simulink model "Final_Model"  (R2013a)
settings: Solver=ode45  StartTime=0.0  StopTime=10.0  RelTol=1e-3
libraries: simulink x47, fuzblock x1
settings Model: Creator=Admin  LastModifiedBy=Admin

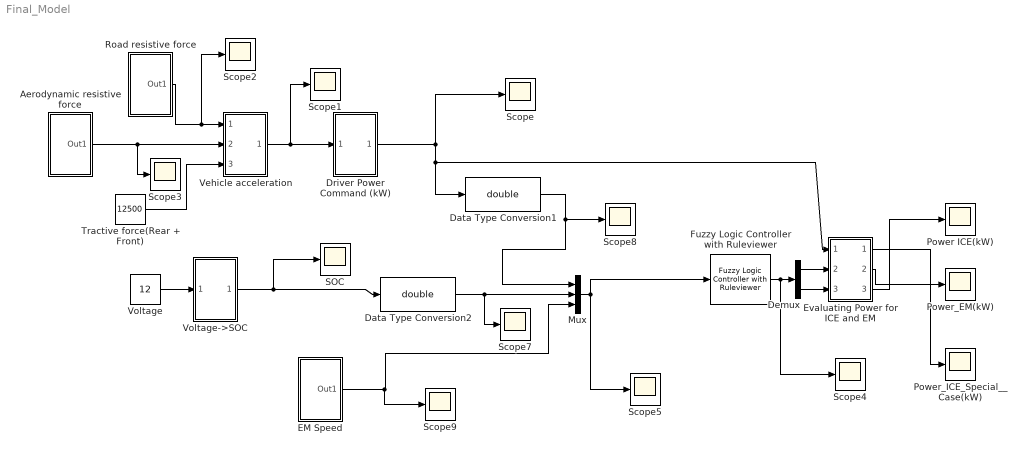
== system Final_Model ==
  Aerodynamic resistive force : Subsystem
  Data Type Conversion1 : DataTypeConversion  OutDataTypeStr=double
  Data Type Conversion2 : DataTypeConversion  OutDataTypeStr=double
  Demux : Demux  Outputs=2
  Driver Power Command (kW) : Subsystem
  EM Speed : Subsystem
  Evaluating Power for ICE and EM : Subsystem
  Fuzzy Logic Controller with Ruleviewer : fuzblock/Fuzzy Logic  Controller  with Ruleviewer  fismatrix=Fuzzy_Controller  Ts=2
  Mux : Mux  Inputs=3
  Power ICE(kW) : Scope
  Power_EM(kW) : Scope
      settings: SaveName=ScopeData6
  Power_ICE_Special__Case(kW) : Scope
      settings: SaveName=ScopeData7
  Road resistive force : Subsystem
  "SOC " : Scope
      settings: SaveName=ScopeData4
  Scope{,1..5,7..9} (9 alike) : Scope
      Scope settings: SaveName=ScopeData5
      Scope1 settings: SaveName=ScopeData8
      Scope2 settings: SaveName=ScopeData9
      Scope3 settings: SaveName=ScopeData10
      Scope4 settings: SaveName=ScopeData11
      Scope5 settings: SaveName=ScopeData2
      Scope7 settings: SaveName=ScopeData14
      Scope8 settings: SaveName=ScopeData15
      Scope9 settings: SaveName=ScopeData3
  Tractive force(Rear + Front) : Constant  Value=12500
  Vehicle acceleration : Subsystem
  Voltage : Constant  Value=12
  Voltage->SOC : Subsystem
  wires:
  Road resistive force/1(Out1) -> Scope2/1, Vehicle acceleration/1(In1)
  Aerodynamic resistive force/1(Out1) -> Scope3/1, Vehicle acceleration/2(In2)
  Tractive force(Rear + Front)/1 -> Vehicle acceleration/3(In3)
  Driver Power Command (kW)/1(Out1) -> Evaluating Power for ICE and EM/1(In1), Data Type Conversion1/1, Scope/1
  EM Speed/1(Out1) -> Scope9/1, Mux/3
  Voltage/1 -> Voltage->SOC/1(In1)
  Fuzzy Logic Controller with Ruleviewer/1 -> Scope4/1, Demux/1
  Mux/1 -> Scope5/1, Fuzzy Logic Controller with Ruleviewer/1
  Data Type Conversion1/1 -> Mux/1, Scope8/1
  Data Type Conversion2/1 -> Scope7/1, Mux/2
  Demux/1 -> Evaluating Power for ICE and EM/2(In2)
  Demux/2 -> Evaluating Power for ICE and EM/3(In3)
  Evaluating Power for ICE and EM/1(Out1) -> Power_ICE_Special__Case(kW)/1
  Evaluating Power for ICE and EM/2(Out2) -> Power_EM(kW)/1
  Voltage->SOC/1(Out1) -> Data Type Conversion2/1, "SOC "/1
  Evaluating Power for ICE and EM/3(Out3) -> Power ICE(kW)/1
  Vehicle acceleration/1(Out1) -> Scope1/1, Driver Power Command (kW)/1(In1)

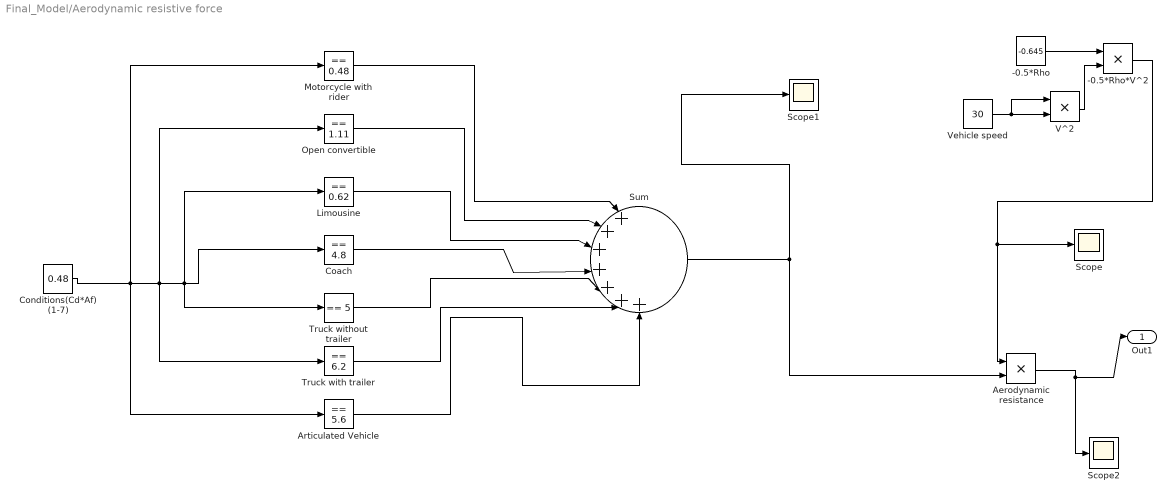
== system Final_Model/Aerodynamic resistive force ==
  -0.5*Rho : Constant  Value=-0.645
  -0.5*Rho*V^2 : Product  RndMeth=Zero
  Aerodynamic resistance : Product  RndMeth=Zero
  Articulated Vehicle : simulink/Logic and Bit Operations/Compare To Constant  relop===  const=5.6  OutDataTypeStr=uint8
  Coach : simulink/Logic and Bit Operations/Compare To Constant  relop===  const=4.8  OutDataTypeStr=uint8
  Conditions(Cd*Af) (1-7) : Constant  Value=0.48
  Limousine : simulink/Logic and Bit Operations/Compare To Constant  relop===  const=0.62  OutDataTypeStr=uint8
  "Motorcycle with rider " : simulink/Logic and Bit Operations/Compare To Constant  relop===  const=0.48  OutDataTypeStr=uint8
  Open convertible : simulink/Logic and Bit Operations/Compare To Constant  relop===  const=1.11  OutDataTypeStr=uint8
  Scope : Scope
      settings: SaveName=ScopeData12
  Scope1 : Scope
      settings: SaveName=ScopeData16
  Scope2 : Scope
      settings: SaveName=ScopeData17
  Sum : Sum  Inputs=|+++++++
  Truck with trailer : simulink/Logic and Bit Operations/Compare To Constant  relop===  const=6.2  OutDataTypeStr=uint8
  Truck without trailer : simulink/Logic and Bit Operations/Compare To Constant  relop===  const=5  OutDataTypeStr=uint8
  V^2 : Product  RndMeth=Zero
  Vehicle speed : Constant  Value=30
  Out1 : Outport
  wires:
  Sum/1 -> Aerodynamic resistance/2, Scope1/1
  Aerodynamic resistance/1 -> Scope2/1, Out1/1
  -0.5*Rho*V^2/1 -> Aerodynamic resistance/1, Scope/1
  V^2/1 -> -0.5*Rho*V^2/2
  -0.5*Rho/1 -> -0.5*Rho*V^2/1
  Conditions(Cd*Af) (1-7)/1 -> "Motorcycle with rider "/1, Articulated Vehicle/1, Open convertible/1, Truck with trailer/1, Limousine/1, Truck without trailer/1, Coach/1
  Truck without trailer/1 -> Sum/5
  Truck with trailer/1 -> Sum/6
  Articulated Vehicle/1 -> Sum/7
  Coach/1 -> Sum/4
  Limousine/1 -> Sum/3
  Open convertible/1 -> Sum/2
  "Motorcycle with rider "/1 -> Sum/1
  Vehicle speed/1 -> V^2/1, V^2/2

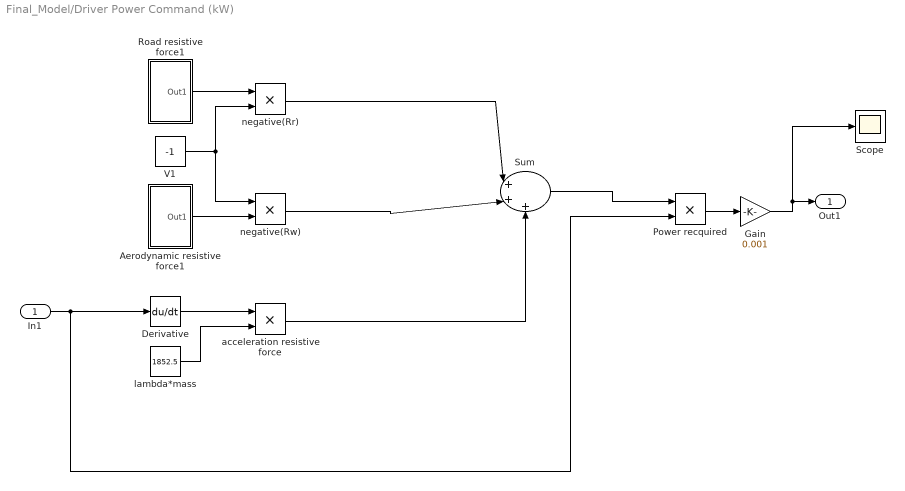
== system Final_Model/Driver Power Command (kW) ==
  In1 : Inport
  Aerodynamic resistive force1 : Subsystem
  Derivative : Derivative
  Gain : Gain  Gain=0.001
  Power recquired : Product  OutDataTypeStr=double  RndMeth=Zero
  Road resistive force1 : Subsystem
  Scope : Scope
      settings: SaveName=ScopeData25
  Sum : Sum  Inputs=|+++  SampleTime=2
  V1 : Constant  Value=-1
  acceleration resistive force : Product  RndMeth=Zero
  lambda*mass : Constant  Value=1852.5
  negative(Rr) : Product  RndMeth=Zero
  negative(Rw) : Product  RndMeth=Zero
  Out1 : Outport
  wires:
  In1/1 -> Power recquired/2, Derivative/1
  Derivative/1 -> acceleration resistive force/1
  lambda*mass/1 -> acceleration resistive force/2
  Road resistive force1/1(Out1) -> negative(Rr)/1
  V1/1 -> negative(Rw)/1, negative(Rr)/2
  Aerodynamic resistive force1/1(Out1) -> negative(Rw)/2
  acceleration resistive force/1 -> Sum/3
  negative(Rw)/1 -> Sum/2
  negative(Rr)/1 -> Sum/1
  Sum/1 -> Power recquired/1
  Power recquired/1 -> Gain/1
  Gain/1 -> Scope/1, Out1/1

== system Final_Model/EM Speed ==
  DC motor : Subsystem
  Out1 : Outport
  wires:
  DC motor/1(Out1) -> Out1/1

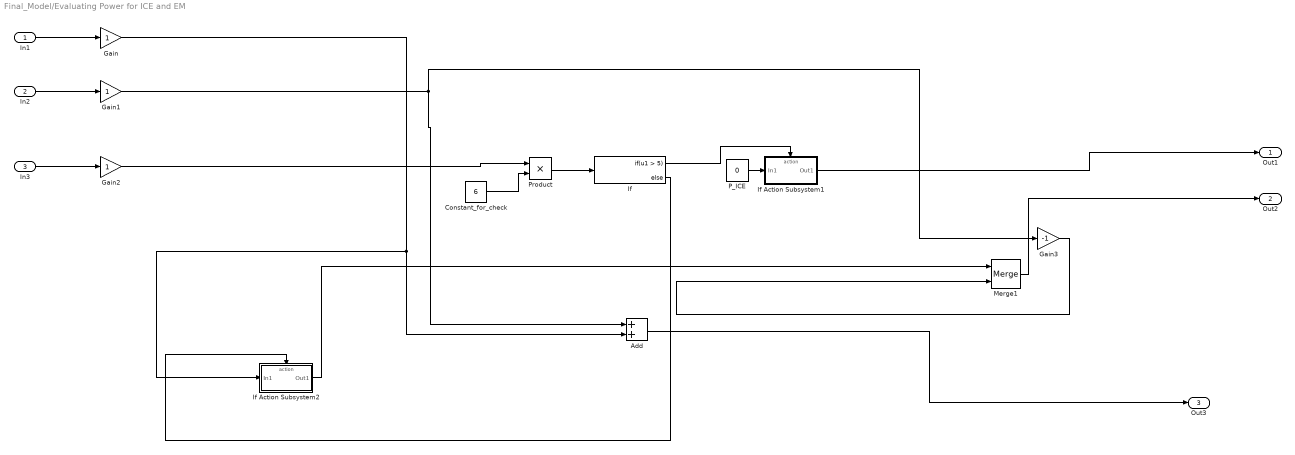
== system Final_Model/Evaluating Power for ICE and EM ==
  In1 : Inport
  In2 : Inport  Port=2
  In3 : Inport  Port=3
  Add : Sum
  Constant_for_check : Constant  Value=6
  Gain : Gain
  Gain1 : Gain
  Gain2 : Gain
  Gain3 : Gain  Gain=-1
  If : If  IfExpression=u1 > 5
  If Action Subsystem1 : Subsystem  TreatAsAtomicUnit=on
  If Action Subsystem2 : Subsystem  TreatAsAtomicUnit=on
  Merge1 : Merge
  P_ICE : Constant  Value=0
  Product : Product
  Out1 : Outport
  Out2 : Outport  Port=2
  Out3 : Outport  Port=3
  wires:
  Merge1/1 -> Out2/1
  Gain3/1 -> Merge1/2
  P_ICE/1 -> If Action Subsystem1/1(In1)
  If/1 -> If Action Subsystem1/Action
  If/2 -> If Action Subsystem2/Action
  Gain/1 -> Add/2, If Action Subsystem2/1(In1)
  In2/1 -> Gain1/1
  In3/1 -> Gain2/1
  Gain2/1 -> Product/1
  Constant_for_check/1 -> Product/2
  Gain1/1 -> Add/1, Gain3/1
  If Action Subsystem2/1(Out1) -> Merge1/1
  In1/1 -> Gain/1
  Product/1 -> If/1
  If Action Subsystem1/1(Out1) -> Out1/1
  Add/1 -> Out3/1

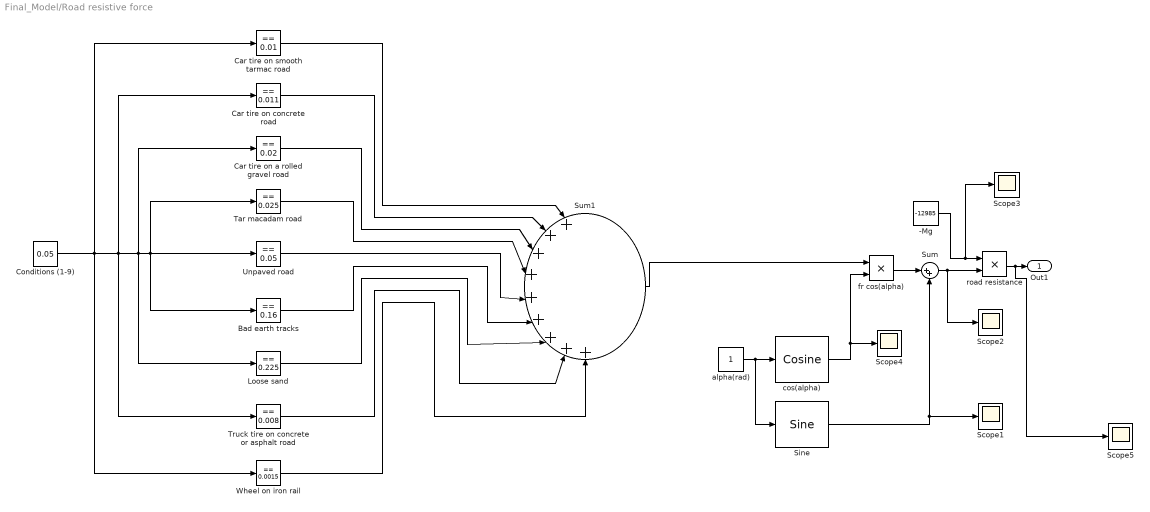
== system Final_Model/Road resistive force ==
  "-Mg " : Constant  Value=-12985
  Bad earth tracks : simulink/Logic and Bit Operations/Compare To Constant  relop===  const=0.16  OutDataTypeStr=uint8
  "Car tire on a rolled gravel road " : simulink/Logic and Bit Operations/Compare To Constant  relop===  const=0.02  OutDataTypeStr=uint8
  Car tire on concrete road : simulink/Logic and Bit Operations/Compare To Constant  relop===  const=0.011  OutDataTypeStr=uint8
  "Car tire on smooth tarmac road " : simulink/Logic and Bit Operations/Compare To Constant  relop===  const=0.01  OutDataTypeStr=uint8
  Conditions (1-9) : Constant  Value=0.05
  Loose sand : simulink/Logic and Bit Operations/Compare To Constant  relop===  const=0.225  OutDataTypeStr=uint8
  Scope{1..5} (5 alike) : Scope
      Scope1 settings: SaveName=ScopeData18
      Scope2 settings: SaveName=ScopeData19
      Scope3 settings: SaveName=ScopeData20
      Scope4 settings: SaveName=ScopeData21
      Scope5 settings: SaveName=ScopeData22
  Sine : simulink/Lookup Tables/Sine  Formula=sin(2*pi*u)  NumDataPoints=(2^5)+1  OutputWordLength=16
  Sum : Sum  Inputs=|++
  Sum1 : Sum  Inputs=|+++++++++
  Tar macadam road : simulink/Logic and Bit Operations/Compare To Constant  relop===  const=0.025  OutDataTypeStr=uint8
  Truck tire on concrete or asphalt road : simulink/Logic and Bit Operations/Compare To Constant  relop===  const=0.008  OutDataTypeStr=uint8
  Unpaved road : simulink/Logic and Bit Operations/Compare To Constant  relop===  const=0.05  OutDataTypeStr=uint8
  Wheel on iron rail : simulink/Logic and Bit Operations/Compare To Constant  relop===  const=0.0015  OutDataTypeStr=uint8
  alpha(rad) : Constant
  cos(alpha) : simulink/Lookup Tables/Cosine  Formula=cos(2*pi*u)  NumDataPoints=(2^5)+1  OutputWordLength=16
  fr cos(alpha) : Product  RndMeth=Zero
  road resistance : Product  RndMeth=Zero
  Out1 : Outport
  wires:
  road resistance/1 -> Scope5/1, Out1/1
  "-Mg "/1 -> Scope3/1, road resistance/1
  Sum/1 -> Scope2/1, road resistance/2
  Sine/1 -> Scope1/1, Sum/2
  fr cos(alpha)/1 -> Sum/1
  alpha(rad)/1 -> Sine/1, cos(alpha)/1
  Sum1/1 -> fr cos(alpha)/1
  cos(alpha)/1 -> Scope4/1, fr cos(alpha)/2
  "Car tire on smooth tarmac road "/1 -> Sum1/1
  Car tire on concrete road/1 -> Sum1/2
  "Car tire on a rolled gravel road "/1 -> Sum1/3
  Tar macadam road/1 -> Sum1/4
  Wheel on iron rail/1 -> Sum1/9
  Truck tire on concrete or asphalt road/1 -> Sum1/8
  Loose sand/1 -> Sum1/7
  Bad earth tracks/1 -> Sum1/6
  Unpaved road/1 -> Sum1/5
  Conditions (1-9)/1 -> Wheel on iron rail/1, Truck tire on concrete or asphalt road/1, Loose sand/1, Bad earth tracks/1, Tar macadam road/1, Unpaved road/1, "Car tire on a rolled gravel road "/1, Car tire on concrete road/1, "Car tire on smooth tarmac road "/1

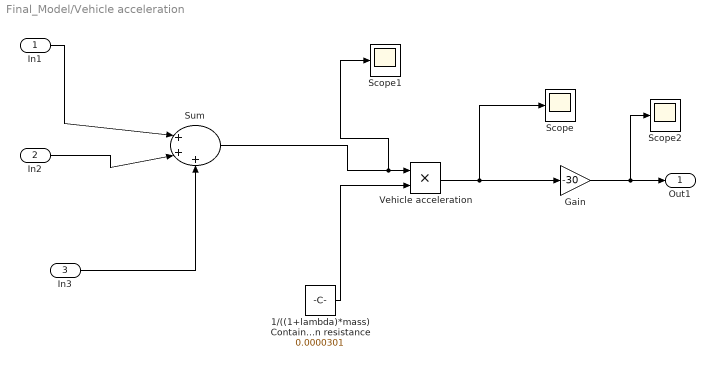
== system Final_Model/Vehicle acceleration ==
  In1 : Inport
  In2 : Inport  Port=2
  In3 : Inport  Port=3
  1/((1+lambda)*mass) Contains acceleration resistance : Constant  Value=0.0000301
  Gain : Gain  Gain=-30
  Scope : Scope
  Scope1 : Scope
      settings: SaveName=ScopeData23
  Scope2 : Scope
      settings: SaveName=ScopeData24
  Sum : Sum  Inputs=|+++
  Vehicle acceleration : Product  RndMeth=Zero
  Out1 : Outport
  wires:
  In1/1 -> Sum/1
  In2/1 -> Sum/2
  In3/1 -> Sum/3
  Sum/1 -> Scope1/1, Vehicle acceleration/1
  1/((1+lambda)*mass) Contains acceleration resistance/1 -> Vehicle acceleration/2
  Vehicle acceleration/1 -> Gain/1, Scope/1
  Gain/1 -> Scope2/1, Out1/1

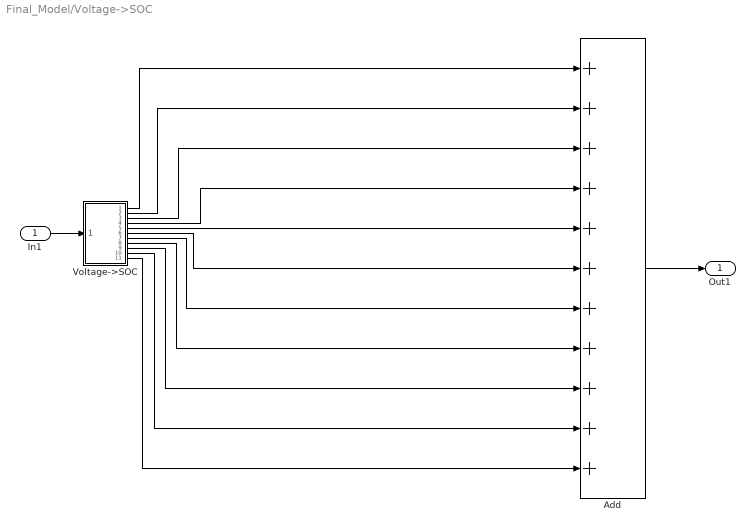
== system Final_Model/Voltage->SOC ==
  In1 : Inport
  Add : Sum  Inputs=+++++++++++  AccumDataTypeStr=uint16  OutDataTypeStr=uint16
  Voltage->SOC : Subsystem
  Out1 : Outport  OutDataTypeStr=uint16
  wires:
  In1/1 -> Voltage->SOC/1(In1)
  Voltage->SOC/1(Out1) -> Add/1
  Voltage->SOC/3(Out3) -> Add/3
  Voltage->SOC/2(Out2) -> Add/2
  Voltage->SOC/10(Out10) -> Add/10
  Voltage->SOC/4(Out4) -> Add/4
  Voltage->SOC/5(Out5) -> Add/5
  Voltage->SOC/6(Out6) -> Add/6
  Voltage->SOC/7(Out7) -> Add/7
  Voltage->SOC/8(Out8) -> Add/8
  Voltage->SOC/9(Out9) -> Add/9
  Add/1 -> Out1/1
  Voltage->SOC/11(Out11) -> Add/11

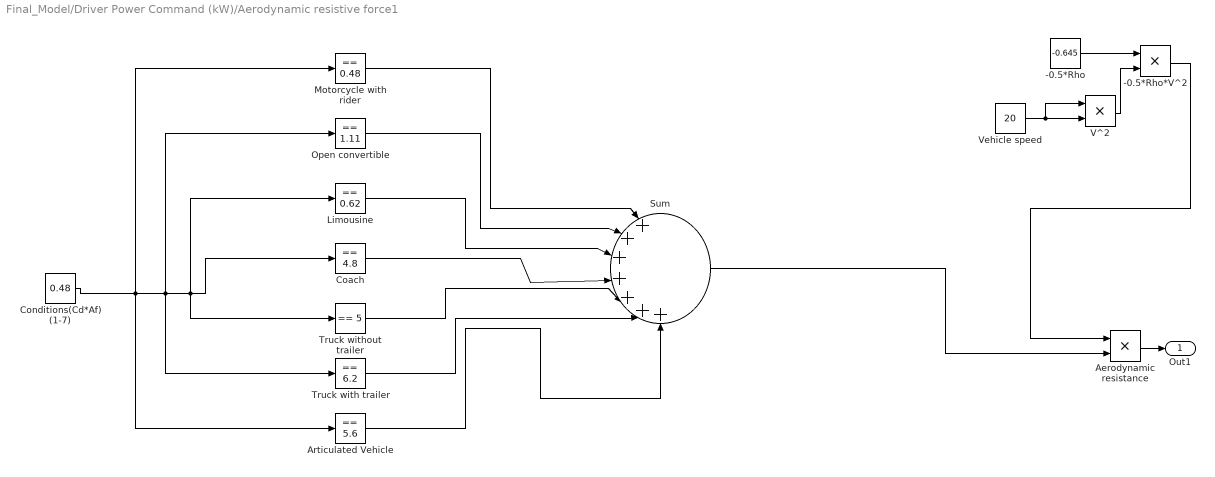
== system Final_Model/Driver Power Command (kW)/Aerodynamic resistive force1 ==
  -0.5*Rho : Constant  Value=-0.645
  -0.5*Rho*V^2 : Product  RndMeth=Zero
  Aerodynamic resistance : Product  RndMeth=Zero
  Articulated Vehicle : simulink/Logic and Bit Operations/Compare To Constant  relop===  const=5.6  OutDataTypeStr=uint8
  Coach : simulink/Logic and Bit Operations/Compare To Constant  relop===  const=4.8  OutDataTypeStr=uint8
  Conditions(Cd*Af) (1-7) : Constant  Value=0.48
  Limousine : simulink/Logic and Bit Operations/Compare To Constant  relop===  const=0.62  OutDataTypeStr=uint8
  "Motorcycle with rider " : simulink/Logic and Bit Operations/Compare To Constant  relop===  const=0.48  OutDataTypeStr=uint8
  Open convertible : simulink/Logic and Bit Operations/Compare To Constant  relop===  const=1.11  OutDataTypeStr=uint8
  Sum : Sum  Inputs=|+++++++
  Truck with trailer : simulink/Logic and Bit Operations/Compare To Constant  relop===  const=6.2  OutDataTypeStr=uint8
  Truck without trailer : simulink/Logic and Bit Operations/Compare To Constant  relop===  const=5  OutDataTypeStr=uint8
  V^2 : Product  RndMeth=Zero
  Vehicle speed : Constant  Value=20
  Out1 : Outport
  wires:
  Sum/1 -> Aerodynamic resistance/2
  Aerodynamic resistance/1 -> Out1/1
  -0.5*Rho*V^2/1 -> Aerodynamic resistance/1
  V^2/1 -> -0.5*Rho*V^2/2
  -0.5*Rho/1 -> -0.5*Rho*V^2/1
  Conditions(Cd*Af) (1-7)/1 -> "Motorcycle with rider "/1, Articulated Vehicle/1, Open convertible/1, Truck with trailer/1, Limousine/1, Truck without trailer/1, Coach/1
  Truck without trailer/1 -> Sum/5
  Truck with trailer/1 -> Sum/6
  Articulated Vehicle/1 -> Sum/7
  Coach/1 -> Sum/4
  Limousine/1 -> Sum/3
  Open convertible/1 -> Sum/2
  "Motorcycle with rider "/1 -> Sum/1
  Vehicle speed/1 -> V^2/1, V^2/2

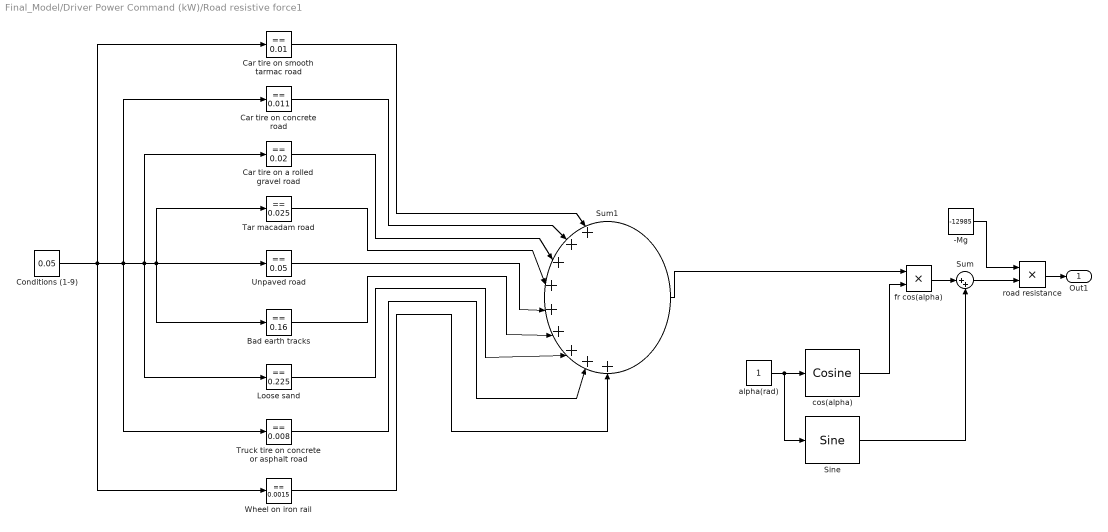
== system Final_Model/Driver Power Command (kW)/Road resistive force1 ==
  "-Mg " : Constant  Value=-12985
  Bad earth tracks : simulink/Logic and Bit Operations/Compare To Constant  relop===  const=0.16  OutDataTypeStr=uint8
  "Car tire on a rolled gravel road " : simulink/Logic and Bit Operations/Compare To Constant  relop===  const=0.02  OutDataTypeStr=uint8
  Car tire on concrete road : simulink/Logic and Bit Operations/Compare To Constant  relop===  const=0.011  OutDataTypeStr=uint8
  "Car tire on smooth tarmac road " : simulink/Logic and Bit Operations/Compare To Constant  relop===  const=0.01  OutDataTypeStr=uint8
  Conditions (1-9) : Constant  Value=0.05
  Loose sand : simulink/Logic and Bit Operations/Compare To Constant  relop===  const=0.225  OutDataTypeStr=uint8
  Sine : simulink/Lookup Tables/Sine  Formula=sin(2*pi*u)  NumDataPoints=(2^5)+1  OutputWordLength=16
  Sum : Sum  Inputs=|++
  Sum1 : Sum  Inputs=|+++++++++
  Tar macadam road : simulink/Logic and Bit Operations/Compare To Constant  relop===  const=0.025  OutDataTypeStr=uint8
  Truck tire on concrete or asphalt road : simulink/Logic and Bit Operations/Compare To Constant  relop===  const=0.008  OutDataTypeStr=uint8
  Unpaved road : simulink/Logic and Bit Operations/Compare To Constant  relop===  const=0.05  OutDataTypeStr=uint8
  Wheel on iron rail : simulink/Logic and Bit Operations/Compare To Constant  relop===  const=0.0015  OutDataTypeStr=uint8
  alpha(rad) : Constant
  cos(alpha) : simulink/Lookup Tables/Cosine  Formula=cos(2*pi*u)  NumDataPoints=(2^5)+1  OutputWordLength=16
  fr cos(alpha) : Product  RndMeth=Zero
  road resistance : Product  RndMeth=Zero
  Out1 : Outport
  wires:
  road resistance/1 -> Out1/1
  "-Mg "/1 -> road resistance/1
  Sum/1 -> road resistance/2
  Sine/1 -> Sum/2
  fr cos(alpha)/1 -> Sum/1
  alpha(rad)/1 -> Sine/1, cos(alpha)/1
  Sum1/1 -> fr cos(alpha)/1
  cos(alpha)/1 -> fr cos(alpha)/2
  "Car tire on smooth tarmac road "/1 -> Sum1/1
  Car tire on concrete road/1 -> Sum1/2
  "Car tire on a rolled gravel road "/1 -> Sum1/3
  Tar macadam road/1 -> Sum1/4
  Wheel on iron rail/1 -> Sum1/9
  Truck tire on concrete or asphalt road/1 -> Sum1/8
  Loose sand/1 -> Sum1/7
  Bad earth tracks/1 -> Sum1/6
  Unpaved road/1 -> Sum1/5
  Conditions (1-9)/1 -> Wheel on iron rail/1, Truck tire on concrete or asphalt road/1, Loose sand/1, Bad earth tracks/1, Tar macadam road/1, Unpaved road/1, "Car tire on a rolled gravel road "/1, Car tire on concrete road/1, "Car tire on smooth tarmac road "/1

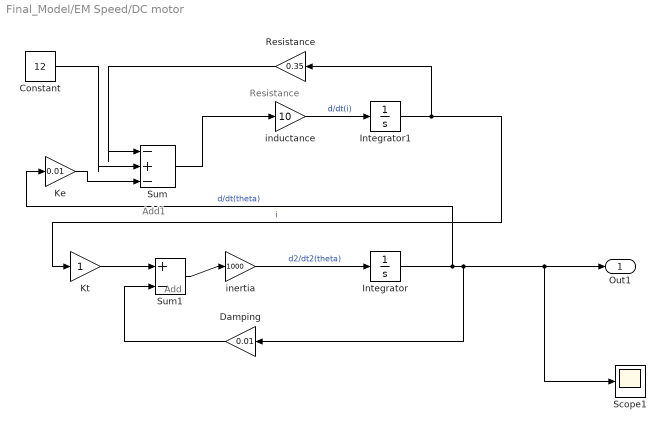
== system Final_Model/EM Speed/DC motor ==
  note: Add1
  note: Add
  note: Resistance
  Constant : Constant  Value=12
  Damping : Gain  Gain=0.01
  Integrator : Integrator
  Integrator1 : Integrator
  Ke : Gain  Gain=0.01
  Kt : Gain
  Resistance : Gain  Gain=0.35
      settings: AttributesFormatString=Resistance
  Scope1 : Scope
      settings: SaveName=ScopeData26
  Sum : Sum  Inputs=|-+-
  Sum1 : Sum  Inputs=|+-
  inductance : Gain  Gain=10
      settings: AttributesFormatString=1/L
  inertia : Gain  Gain=1000
      settings: AttributesFormatString=1/J
  Out1 : Outport
  wires:
  Integrator/1 -> Ke/1, Scope1/1, Out1/1, Damping/1  "d/dt(theta)"
  inductance/1 -> Integrator1/1  "d/dt(i)"
  Sum/1 -> inductance/1
  Resistance/1 -> Sum/1
  Ke/1 -> Sum/3
  Integrator1/1 -> Kt/1, Resistance/1  "i"
  inertia/1 -> Integrator/1  "d2/dt2(theta)"
  Sum1/1 -> inertia/1
  Damping/1 -> Sum1/2
  Kt/1 -> Sum1/1
  Constant/1 -> Sum/2

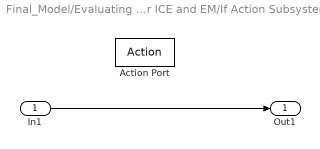
== system Final_Model/Evaluating Power for ICE and EM/If Action Subsystem1 ==
  In1 : Inport
  Action Port : ActionPort  ActionType=then
  Out1 : Outport
  wires:
  In1/1 -> Out1/1

== system Final_Model/Evaluating Power for ICE and EM/If Action Subsystem2 ==
  In1 : Inport
  Action Port : ActionPort  ActionType=else
  Out1 : Outport
  wires:
  In1/1 -> Out1/1

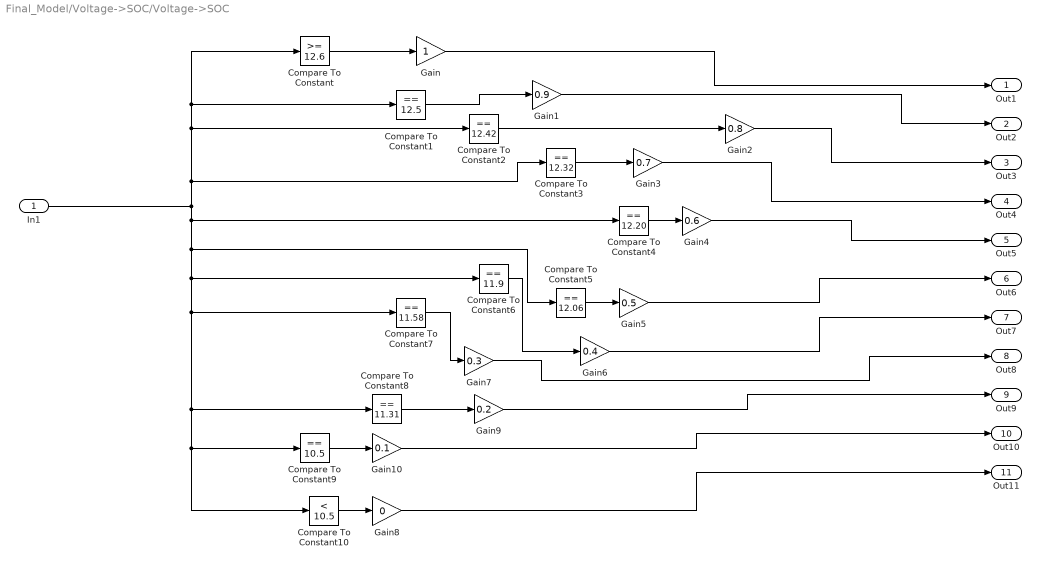
== system Final_Model/Voltage->SOC/Voltage->SOC ==
  In1 : Inport
  Compare To Constant : simulink/Logic and Bit Operations/Compare To Constant  relop=>=  const=12.6  OutDataTypeStr=uint8  ZeroCross=off
  Compare To Constant1 : simulink/Logic and Bit Operations/Compare To Constant  relop===  const=12.5  OutDataTypeStr=uint8  ZeroCross=off
  Compare To Constant10 : simulink/Logic and Bit Operations/Compare To Constant  relop=<  const=10.5  OutDataTypeStr=uint8
  Compare To Constant2 : simulink/Logic and Bit Operations/Compare To Constant  relop===  const=12.42  OutDataTypeStr=uint8
  Compare To Constant3 : simulink/Logic and Bit Operations/Compare To Constant  relop===  const=12.32  OutDataTypeStr=uint8
  Compare To Constant4 : simulink/Logic and Bit Operations/Compare To Constant  relop===  const=12.20  OutDataTypeStr=uint8
  Compare To Constant5 : simulink/Logic and Bit Operations/Compare To Constant  relop===  const=12.06  OutDataTypeStr=uint8
  Compare To Constant6 : simulink/Logic and Bit Operations/Compare To Constant  relop===  const=11.9  OutDataTypeStr=uint8
  Compare To Constant7 : simulink/Logic and Bit Operations/Compare To Constant  relop===  const=11.58  OutDataTypeStr=uint8
  Compare To Constant8 : simulink/Logic and Bit Operations/Compare To Constant  relop===  const=11.31  OutDataTypeStr=uint8
  Compare To Constant9 : simulink/Logic and Bit Operations/Compare To Constant  relop===  const=10.5  OutDataTypeStr=uint8
  Gain : Gain
  Gain1 : Gain  Gain=0.9
  Gain10 : Gain  Gain=0.1
  Gain2 : Gain  Gain=0.8
  Gain3 : Gain  Gain=0.7
  Gain4 : Gain  Gain=0.6
  Gain5 : Gain  Gain=0.5
  Gain6 : Gain  Gain=0.4
  Gain7 : Gain  Gain=0.3
  Gain8 : Gain  Gain=0
  Gain9 : Gain  Gain=0.2
  Out1 : Outport
  Out2 : Outport  Port=2
  Out3 : Outport  Port=3
  Out4 : Outport  Port=4
  Out5 : Outport  Port=5
  Out6 : Outport  Port=6
  Out7 : Outport  Port=7
  Out8 : Outport  Port=8
  Out9 : Outport  Port=9
  Out10 : Outport  Port=10
  Out11 : Outport  Port=11
  wires:
  Gain8/1 -> Out11/1
  Gain10/1 -> Out10/1
  Gain9/1 -> Out9/1
  Gain7/1 -> Out8/1
  Gain6/1 -> Out7/1
  Gain5/1 -> Out6/1
  Gain4/1 -> Out5/1
  Gain3/1 -> Out4/1
  Gain2/1 -> Out3/1
  Gain1/1 -> Out2/1
  Gain/1 -> Out1/1
  Compare To Constant10/1 -> Gain8/1
  Compare To Constant9/1 -> Gain10/1
  Compare To Constant8/1 -> Gain9/1
  Compare To Constant7/1 -> Gain7/1
  Compare To Constant6/1 -> Gain6/1
  Compare To Constant5/1 -> Gain5/1
  Compare To Constant4/1 -> Gain4/1
  Compare To Constant3/1 -> Gain3/1
  Compare To Constant2/1 -> Gain2/1
  Compare To Constant1/1 -> Gain1/1
  Compare To Constant/1 -> Gain/1
  In1/1 -> Compare To Constant3/1, Compare To Constant/1, Compare To Constant1/1, Compare To Constant2/1, Compare To Constant4/1, Compare To Constant5/1, Compare To Constant7/1, Compare To Constant10/1, Compare To Constant9/1, Compare To Constant8/1, Compare To Constant6/1
